simulink model "Dynamic_mini_project_b"  (R2022b)
settings: Solver=VariableStepAuto  StartTime=0.0  StopTime=10  FixedStep=0.1  MaxStep=0.002  RelTol=1e-3
settings Model: Creator=Jakob Jørgensen  LastModifiedBy=Jakob Jørgensen

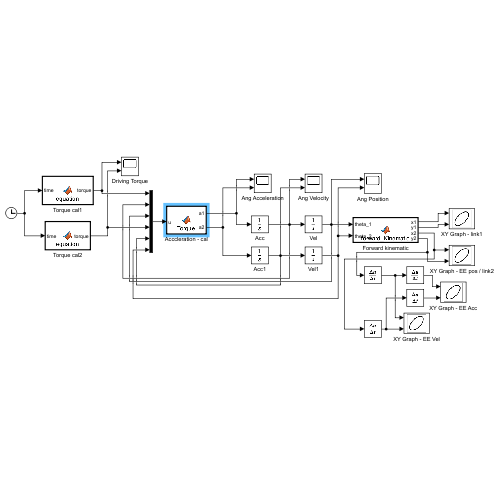
[thumbnail: Simulink's stored preview of the top-level diagram]
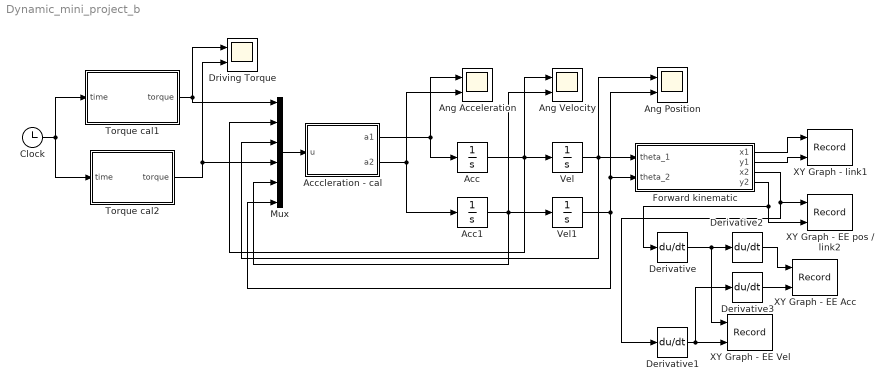
== system Dynamic_mini_project_b ==
  Acc : Integrator
  Acc1 : Integrator
  Acccleration - cal : MATLAB Function  TreatAsAtomicUnit=on
  Ang Acceleration : Scope  NumInputPorts=2
  Ang Position : Scope  NumInputPorts=2
  Ang Velocity : Scope  NumInputPorts=2
  Clock : Clock
  Derivative{,1..3} (4 alike) : Derivative
  Driving Torque : Scope  NumInputPorts=2
  Forward kinematic : MATLAB Function  TreatAsAtomicUnit=on
  Mux : Mux  Inputs=6
  Torque cal1 : MATLAB Function  TreatAsAtomicUnit=on
  Torque cal2 : MATLAB Function  TreatAsAtomicUnit=on
  Vel : Integrator
  Vel1 : Integrator
  XY Graph - EE Acc : Record  FileSettingsInternal="{\"entries\":[{\"content\":{\"excelSettings\":{\"content\":{},\"type\":\"Streamout.ExcelSettings\"}},\"type\":\"Streamout.FileSettingStorage\",\"uuid\":\"9bbb8e30-f031-4086-aa11-3c3b12b71465\"}],\"packageUris\":[\"http://schema.mathworks.com/mf0/streamout_blocks/R2020a\"],\"version\":\"1.0\"}"  Layout=[1 1]  SignalsInternal="{\"entries\":[{\"content\":{\"signals\":[{\"content\":{\"blockPath\":[\"Dynamic_mini_project_b/XY Graph - EE Acc\"],\"channel\":[],\"dimensions\":[1],\"domain\":\"Dynamic_mini_project_b/XY Graph - EE Acc\",\"lineColor\":\"#edb120\",\"plots\":[1],\"port\":1,\"sid\":[\"\"],\"signalID\":1051,\"signalName\":\"Derivative2\"},\"type\":\"RecordBlkView.Signal\",\"uuid\":\"09e1cdd4-9cc9-4b86-bc8d-48142a0b626b\"},{\"content\":{\"blockPath\":[\"Dynamic_mini_project_b/XY Graph - EE Acc\"],\"channel\":[],\"dimensions\":[1],\"domain\":\"Dynamic_mini_project_b/XY Graph - EE Acc\",\"lineColor\":\"#7e2f8e\",\"plots\":[1],\"port\":2,\"sid\":[\"\"],\"signalID\":1055,\"signalName\":\"Derivative3\"},\"type\":\"RecordBlkView.Signal\",\"uuid\":\"62cbbc6e-7952-47fe-a8b0-100ed0d424dc\"}]},\"type\":\"RecordBlkView.InputSignals\",\"uuid\":\"a32a90c5-a282-40a4-ac00-918dc37c2d35\"}],\"packageUris\":[\"http://schema.mathworks.com/mf0/streamout_blocks/R2020a\"],\"version\":\"1.0\"}"  VisualizationBindings="{\"xyplotplugin\":{\"info\":[{\"series\":[{\"bindingParametersList\":[{\"parameter\":\"X-Axis\",\"signalID\":1051,\"signalName\":\"Derivative2\"},{\"parameter\":\"Y-Axis\",\"signalID\":1055,\"signalName\":\"Derivative3\"}],\"seriesID\":348}],\"subplotID\":1}]}}"  CompatibilityTag=XY
  XY Graph - EE Vel : Record  FileSettingsInternal="{\"entries\":[{\"content\":{\"excelSettings\":{\"content\":{},\"type\":\"Streamout.ExcelSettings\"}},\"type\":\"Streamout.FileSettingStorage\",\"uuid\":\"188ebd1f-119c-4b44-81ae-267975c8f331\"}],\"packageUris\":[\"http://schema.mathworks.com/mf0/streamout_blocks/R2020a\"],\"version\":\"1.0\"}"  Layout=[1 1]  SignalsInternal="{\"entries\":[{\"content\":{\"signals\":[{\"content\":{\"blockPath\":[\"Dynamic_mini_project_b/XY Graph - EE Vel\"],\"channel\":[],\"dimensions\":[1],\"domain\":\"Dynamic_mini_project_b/XY Graph - EE Vel\",\"lineColor\":\"#77ac30\",\"plots\":[1],\"port\":1,\"sid\":[\"\"],\"signalID\":1059,\"signalName\":\"Derivative\"},\"type\":\"RecordBlkView.Signal\",\"uuid\":\"b0c24f2f-c17e-4899-a181-925681eb8237\"},{\"content\":{\"blockPath\":[\"Dynamic_mini_project_b/XY Graph - EE Vel\"],\"channel\":[],\"dimensions\":[1],\"domain\":\"Dynamic_mini_project_b/XY Graph - EE Vel\",\"lineColor\":\"#4dbeee\",\"plots\":[1],\"port\":2,\"sid\":[\"\"],\"signalID\":1063,\"signalName\":\"Derivative1\"},\"type\":\"RecordBlkView.Signal\",\"uuid\":\"44dcd9bf-f71d-481e-b018-710e022d5d2f\"}]},\"type\":\"RecordBlkView.InputSignals\",\"uuid\":\"94f1331b-6e45-4ea8-8e93-5714a4349c40\"}],\"packageUris\":[\"http://schema.mathworks.com/mf0/streamout_blocks/R2020a\"],\"version\":\"1.0\"}"  VisualizationBindings="{\"xyplotplugin\":{\"info\":[{\"series\":[{\"bindingParametersList\":[{\"parameter\":\"X-Axis\",\"signalID\":1059,\"signalName\":\"Derivative\"},{\"parameter\":\"Y-Axis\",\"signalID\":1063,\"signalName\":\"Derivative1\"}],\"seriesID\":668}],\"subplotID\":1}]}}"  CompatibilityTag=XY
  XY Graph - EE pos / link2 : Record  FileSettingsInternal="{\"entries\":[{\"content\":{\"excelSettings\":{\"content\":{},\"type\":\"Streamout.ExcelSettings\"}},\"type\":\"Streamout.FileSettingStorage\",\"uuid\":\"42983a66-81c1-4eae-9f3e-4c9c5ebf532b\"}],\"packageUris\":[\"http://schema.mathworks.com/mf0/streamout_blocks/R2020a\"],\"version\":\"1.0\"}"  Layout=[1 1]  SignalsInternal="{\"entries\":[{\"content\":{\"signals\":[{\"content\":{\"blockPath\":[\"Dynamic_mini_project_b/XY Graph - EE pos // link2\"],\"channel\":[],\"dimensions\":[1],\"domain\":\"Dynamic_mini_project_b/XY Graph - EE pos // link2\",\"lineColor\":\"#a2142f\",\"plots\":[1],\"port\":1,\"sid\":[\"\"],\"signalID\":1067,\"signalName\":\"Forward kinematic:3\"},\"type\":\"RecordBlkView.Signal\",\"uuid\":\"87d81417-78a1-459c-8aed-974f46b7f4b4\"},{\"content\":{\"blockPath\":[\"Dynamic_mini_project_b/XY Graph - EE pos // link2\"],\"channel\":[],\"dimensions\":[1],\"domain\":\"Dynamic_mini_project_b/XY Graph - EE pos // link2\",\"lineColor\":\"#139fff\",\"plots\":[1],\"port\":2,\"sid\":[\"\"],\"signalID\":1071,\"signalName\":\"Forward kinematic:4\"},\"type\":\"RecordBlkView.Signal\",\"uuid\":\"836bf671-0a82-4259-bfc5-2a72af552d6c\"}]},\"type\":\"RecordBlkView.InputSignals\",\"uuid\":\"6101818b-3f92-4380-adf0-6adefaac0ac8\"}],\"packageUris\":[\"http://schema.mathworks.com/mf0/streamout_blocks/R2020a\"],\"version\":\"1.0\"}"  VisualizationBindings="{\"xyplotplugin\":{\"info\":[{\"series\":[{\"bindingParametersList\":[{\"parameter\":\"X-Axis\",\"signalID\":1067,\"signalName\":\"Forward kinematic:3\"},{\"parameter\":\"Y-Axis\",\"signalID\":1071,\"signalName\":\"Forward kinematic:4\"}],\"seriesID\":15}],\"subplotID\":1}]}}"  CompatibilityTag=XY
  XY Graph - link1 : Record  FileSettingsInternal="{\"entries\":[{\"content\":{\"excelSettings\":{\"content\":{},\"type\":\"Streamout.ExcelSettings\"}},\"type\":\"Streamout.FileSettingStorage\",\"uuid\":\"d2c7d847-4cb1-4e92-a3c0-13405567ddaa\"}],\"packageUris\":[\"http://schema.mathworks.com/mf0/streamout_blocks/R2020a\"],\"version\":\"1.0\"}"  Layout=[1 1]  SignalsInternal="{\"entries\":[{\"content\":{\"signals\":[{\"content\":{\"blockPath\":[\"Dynamic_mini_project_b/XY Graph - link1\"],\"channel\":[],\"dimensions\":[1],\"domain\":\"Dynamic_mini_project_b/XY Graph - link1\",\"lineColor\":\"#64d413\",\"plots\":[1],\"port\":1,\"sid\":[\"\"],\"signalID\":1075,\"signalName\":\"Forward kinematic:1\"},\"type\":\"RecordBlkView.Signal\",\"uuid\":\"495f6ef1-aec4-4d75-be76-3070379fe138\"},{\"content\":{\"blockPath\":[\"Dynamic_mini_project_b/XY Graph - link1\"],\"channel\":[],\"dimensions\":[1],\"domain\":\"Dynamic_mini_project_b/XY Graph - link1\",\"lineColor\":\"#ff13a6\",\"plots\":[1],\"port\":2,\"sid\":[\"\"],\"signalID\":1079,\"signalName\":\"Forward kinematic:2\"},\"type\":\"RecordBlkView.Signal\",\"uuid\":\"e203565c-3409-47ac-b2cb-3549c10538ce\"}]},\"type\":\"RecordBlkView.InputSignals\",\"uuid\":\"215b2acc-5007-437e-bf1e-15fbecaa8bdb\"}],\"packageUris\":[\"http://schema.mathworks.com/mf0/streamout_blocks/R2020a\"],\"version\":\"1.0\"}"  VisualizationBindings="{\"xyplotplugin\":{\"info\":[{\"series\":[{\"bindingParametersList\":[{\"parameter\":\"X-Axis\",\"signalID\":1075,\"signalName\":\"Forward kinematic:1\"},{\"parameter\":\"Y-Axis\",\"signalID\":1079,\"signalName\":\"Forward kinematic:2\"}],\"seriesID\":34599}],\"subplotID\":1}]}}"  CompatibilityTag=XY
  wires:
  Vel1/1 -> Ang Position/2, Forward kinematic/2(theta_2), Mux/6
  Acc1/1 -> Vel1/1, Mux/5, Ang Velocity/2
  Mux/1 -> Acccleration - cal/1(u)
  Acccleration - cal/2(a2) -> Ang Acceleration/2, Acc1/1
  Acc/1 -> Vel/1, Ang Velocity/1, Mux/2
  Acccleration - cal/1(a1) -> Acc/1, Ang Acceleration/1
  Vel/1 -> Ang Position/1, Forward kinematic/1(theta_1), Mux/3
  Clock/1 -> Torque cal2/1(time), Torque cal1/1(time)
  Torque cal1/1(torque) -> Driving Torque/1, Mux/1
  Torque cal2/1(torque) -> Driving Torque/2, Mux/4
  Forward kinematic/2(y1) -> XY Graph - link1/2
  Forward kinematic/1(x1) -> XY Graph - link1/1
  Forward kinematic/3(x2) -> Derivative1/1, XY Graph - EE pos / link2/1
  Forward kinematic/4(y2) -> XY Graph - EE pos / link2/2, Derivative/1
  Derivative/1 -> Derivative2/1, XY Graph - EE Vel/1
  Derivative1/1 -> Derivative3/1, XY Graph - EE Vel/2
  Derivative2/1 -> XY Graph - EE Acc/1
  Derivative3/1 -> XY Graph - EE Acc/2

== matlab function Dynamic_mini_project_b/Torque cal1 ==
  data: time input; torque output
function torque = equation(time)

if time < 3
    torque = time*2;
elseif time < 6    
    torque= -2*time+12; 
else
    torque = 0;
end

== matlab function Dynamic_mini_project_b/Torque cal2 ==
  data: time input; torque output
function torque = equation(time)

if time < 3
    torque = time*1.166;
elseif time < 6    
    torque= -1.166*time+7; 
else
    torque = 0;
end

== matlab function Dynamic_mini_project_b/Acccleration - cal ==
  data: u input; a1 output; a2 output
function [a1, a2]= Torque(u)

%%   motor torques
tau_1 = u(1);
tau_2 = u(4); 
tau =[tau_1 tau_2];

%% joint velocity and displacement
 theta_1 = u(3);  theta_2 = u(6);
 d_theta_2 =u(5);d_theta_1 = u(2); 

%%  %%%%%%%%%%%%%%%%%%%%%%%  motion profiles
% %=======================  joint 1
% A1 = 0.3; % magnitude
% f1 = 5; % frequency
% 
% %=======================  joint 2
% A2 = 0.5; % magnitude
% f2 = 2; % frequency

g = 9.801; % gravity constant 
rho = 7806; 
%% %%%%%%%%%%%%%%%%%%%%%%%%%%%%  link 1 properties
%======================================  link 1
L1 = 1; % length [m]
c1 = L1/2; % mass center
m1 = L1*0.05*0.05*rho; % mass [kg]
I1 = 1/12*m1*L1^2; % moment of inertia


%% %%%%%%%%%%%%%%%%%%%%%%%%%%%%  link 2 properties
%======================================  link 2
L2 = 0.5; % length [m]
c2 = L2/2; % mass center
m2 = L2*0.05*0.05*rho; % mass [kg] 
%m2 = 0.1;
I2 = 1/12*m2*L2^2; % moment of inertia

%% %%%%%%%%%%%%%%%%%% dynamic simulation

    %%%%%%%%%%%%%%%%%%%%%%%%%%%  coefficients of dynamic equation
    H1 = m1*c1^2 + I1+I2+m2*(L1^2+c2^2+2*L1*c2*cos(theta_2)); 
    H2 = m1*c2^2+I2; 
    H12 = m2*(c2^2+2*L1*c2*cos(theta_2))+I2; 
    h = m2*L1*c2*sin(theta_2); 
    M = [H1 H12;H12 H2]; 

    G1 = m1*g*(c1*cos(theta_1))+m2*g*(L1*cos(theta_1)+c2*cos(theta_1+theta_2));
    G2 = m1*c1*g*cos(theta_1+theta_2);   
    G=[G1 G2]; 

    v_1= -h*d_theta_2^2-2*h*d_theta_1*d_theta_2; 
    v_2=h*d_theta_1^2;
    v= [ v_1 v_2 ];
%actuator accelration
%     tau_1 = H11*ddtheta_1 + H12*ddtheta_2 - h*(dtheta_2)^2 ...
%         -2*h*dtheta_1*dtheta_2 + G1;
%     tau_2 = H22*ddtheta_2 + H12*ddtheta_1 + h*(dtheta_1)^2 + G2;   

a= inv(M).*(tau-(v+G)) ;
a1=a(1);
a2=a(2);

== matlab function Dynamic_mini_project_b/Forward kinematic ==
  data: theta_1 input; x1 output; y1 output; theta_2 input; x2 output; y2 output
function [x1, y1,x2,y2]=  forward_Kinematic(theta_1, theta_2)

l1 = 1;
l2 = 0.5;
x1 = l1*cos(theta_1);
y1 = l1*sin(theta_1);
x2 = l2*cos(theta_1+theta_2) +x1;
y2 = l2*sin(theta_1+theta_2)+ y1;
